simulink model "fuzzy_PI"  (R2019a)
settings: Solver=ode3  StartTime=0.0  StopTime=10.0  FixedStep=Ts  RelTol=1e-3  EnableMultiTasking=on
values from neighbouring files (symbols this model uses):
  K = 24    [fuzzy_gains.m]    (also in task1.m; task2.m; task3.m = 10)
  Kd = a*Ke    (= 0.10952970297)    [fuzzy_gains.m]    (also in task1.m = 0.1095; task2.m = 0.1095; task3.m = 0.0146)
  Ke = 1.5    [fuzzy_gains.m]    (also in task1.m; task2.m; task3.m = 0.2)
  Ts = 0.01    [task1.m]    (also in task2.m; task3.m)
libraries: fuzblock x1
settings Model: Creator=chris  LastModifiedBy=MAG@S
settings DataIOCC: LimitDataPoints=on  SaveFormat=Array
settings OptimizationCC: LifeSpan=inf
settings DebuggingCC: SFUnexpectedBacktrackingDiag=warning  SFNoUnconditionalDefaultTransitionDiag=warning  SFExecutionAtInitializationDiag=none  ArithmeticOperatorsInVariantConditions=warning
settings HardwareCC: ProdBitPerPointer=32  ProdBitPerSizeT=32  ProdBitPerPtrDiffT=32  ProdLargestAtomicFloat=None  ProdIntDivRoundTo=Undefined  ProdEndianess=Unspecified  ProdWordSize=32  ProdHWDeviceType=32-bit Generic
settings ModelReferenceCC: PropagateSignalLabelsOutOfModel=off
settings SFSimCC: SimUseLocalCustomCode=off
settings RTWCC: RTWUseLocalCustomCode=off
settings CodeAppCC: StateflowObjectComments=on
settings GRTTargetCC: TargetLangStandard=C89/C90 (ANSI)  GeneratePreprocessorConditionals=Disable all
settings ConfigComp: CovMetricSettings=dw  CovHtmlReporting=on  CovSaveCumulativeToWorkspaceVar=on  CovSaveSingleToWorkspaceVar=on  CovExternalEMLEnable=off

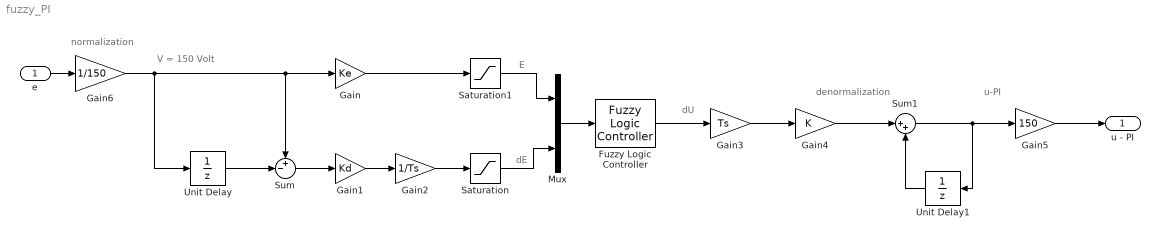
== system fuzzy_PI ==
  note: u-PI
  note: denormalization
  note: normalization
  note: dE
  note: E
  note: dU
  note: V = 150 Volt
  e : Inport
  Fuzzy Logic Controller : fuzblock/Fuzzy Logic  Controller  FIS='fuzzy_motor.fis'  OutputSampleNumber=101  DataType=double  FuzzifiedInputs=off  RuleFiringStrengths=off  RuleOutputs=off  AggregatedOutputs=off  SimulateUsing=Interpreted execution  OutOfRangeInputValueMessage=warning  NoRuleFiredMessage=warning  EmptyOutputFuzzySetMessage=warning
  Gain : Gain  Gain=Ke
  Gain1 : Gain  Gain=Kd
  Gain2 : Gain  Gain=1/Ts
  Gain3 : Gain  Gain=Ts
  Gain4 : Gain  Gain=K
  Gain5 : Gain  Gain=150
  Gain6 : Gain  Gain=1/150
  Mux : Mux  Inputs=2
  Saturation : Saturate  UpperLimit=1  LowerLimit=-1
  Saturation1 : Saturate  UpperLimit=1  LowerLimit=-1
  Sum : Sum  Inputs=+-|
  Sum1 : Sum  Inputs=|++
  Unit Delay : UnitDelay  SampleTime=-1  HasFrameUpgradeWarning=on
  Unit Delay1 : UnitDelay  SampleTime=-1  HasFrameUpgradeWarning=on
  "u - PI " : Outport
  wires:
  e/1 -> Gain6/1
  Unit Delay/1 -> Sum/2
  Sum/1 -> Gain1/1
  Gain1/1 -> Gain2/1
  Gain2/1 -> Saturation/1
  Gain/1 -> Saturation1/1
  Saturation/1 -> Mux/2
  Saturation1/1 -> Mux/1
  Mux/1 -> Fuzzy Logic Controller/1
  Fuzzy Logic Controller/1 -> Gain3/1
  Gain3/1 -> Gain4/1
  Gain6/1 -> Gain/1, Sum/1, Unit Delay/1
  Gain4/1 -> Sum1/1
  Sum1/1 -> Gain5/1, Unit Delay1/1
  Unit Delay1/1 -> Sum1/2
  Gain5/1 -> "u - PI "/1
